simulink model "Calculator"  (R2021a)
settings: Solver=FixedStepDiscrete  StartTime=0.0  StopTime=10.0  RelTol=1e-3  EnableMultiTasking=on
settings Model: Creator=elkny  LastModifiedBy=elkny
settings DataIOCC: ReturnWorkspaceOutputs=off
settings OptimizationCC: DefaultParameterBehavior=Inlined  InlineInvariantSignals=on  EnableMemcpy=off  LifeSpan=1  EfficientTunableParamExpr=on
settings DebuggingCC: UnderspecifiedInitializationDetection=Classic  MergeDetectMultiDrivingBlocksExec=none  SFMachineParentedDataDiag=warning  ArithmeticOperatorsInVariantConditions=warning
settings ModelReferenceCC: PropagateSignalLabelsOutOfModel=off
settings SFSimCC: MATLABDynamicMemAlloc=off  CustomCodeUndefinedFunction=UseInterfaceOnly
settings RTWCC: SystemTargetFile=ert.tlc  GenCodeOnly=on  TemplateMakefile=ert_default_tmf  GenerateReport=on  IncludeHyperlinkInReport=on  LaunchReport=on  GenerateTraceInfo=on  GenerateTraceReport=on  GenerateTraceReportSl=on  GenerateTraceReportSf=on  GenerateTraceReportEml=on
settings CodeAppCC: ForceParamTrailComments=on  IgnoreCustomStorageClasses=off  OperatorAnnotations=on  SimulinkDataObjDesc=on  SFDataObjDesc=on  MATLABFcnDesc=on  InsertBlockDesc=on  StateflowObjectComments=on  MATLABSourceComments=on
settings ERTTargetCC: MultiwordLength=2048  GenerateSampleERTMain=on  InlinedParameterPlacement=NonHierarchical  ERTCustomFileTemplate=example_file_process.tlc

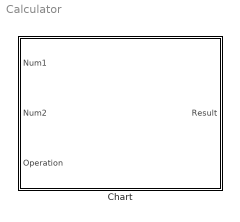
== system Calculator ==
  Chart : Stateflow chart  TreatAsAtomicUnit=on

== stateflow chart Calculator/Chart ==
  state Add(N1,N2) [function]
    (default) -> (junction 48) : {Result=N1+N2;}
  state Sub(N1,N2) [function]
    (default) -> (junction 50) : {Result=N1-N2;}
  state Multiply(N1,N2) [function]
    (default) -> (junction 53) : {Result=N1*N2;}
  state Divide(N1,N2) [function]
    (default) -> (junction 56)
    (junction 56) -> (junction 70) [order 1] : [N2==0]
    (junction 70) -> (junction 72) : {Result=-1}
    (junction 56) -> (junction 72) [order 2] : {Result=N1/N2;}
  (default) -> (junction 36) : % Calculator
  (junction 36) -> (junction 37) [order 1] : [Operation==0]
  (junction 36) -> (junction 38) [order 2]
  (junction 37) -> (junction 45) : {Add(Num1,Num2);}
  (junction 38) -> (junction 39) [order 1] : [Operation==1]
  (junction 38) -> (junction 40) [order 2]
  (junction 39) -> (junction 44) : {Sub(Num1,Num2);}
  (junction 40) -> (junction 41) [order 1] : [Operation==2]
  (junction 40) -> (junction 42) [order 2] : {Divide(Num1,Num2);}
  (junction 41) -> (junction 43) : {Multiply(Num1,Num2);}
  (junction 43) -> (junction 42)
  (junction 44) -> (junction 43)
  (junction 45) -> (junction 44)
  (junction 42) -> (junction 46)
  data: N1 function_input; N2 function_input; N1 function_input; N2 function_input; N1 function_input; N2 function_input; N1 function_input; N2 function_input; Num1 input; Num2 input; Operation input; Result output
